simulink model "sl_onelink_control"  (R2017a)
settings: Solver=VariableStepAuto  StartTime=0.0  StopTime=10.0  RelTol=1e-3
libraries: roblocks x2
settings Model: Creator=mkillpack  LastModifiedBy=mkillpack

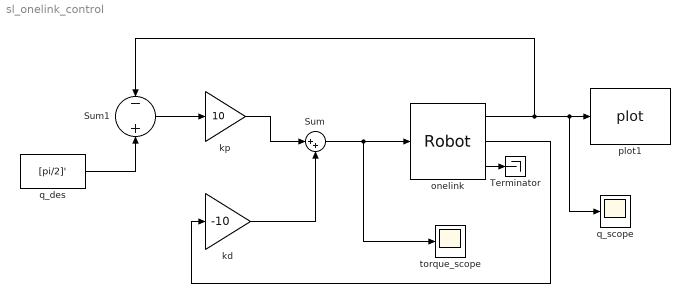
== system sl_onelink_control ==
  Sum : Sum  Inputs=|++
  Sum1 : Sum  Inputs=-|+
  Terminator : Terminator
  kd : Gain  Gain=-10
  kp : Gain  Gain=10
  "onelink " : roblocks/Arm/Robot  robot=onelink  q0=[0]
  plot1 : roblocks/Arm/plot  robot=onelink  fps=10  holdplot=on
  q_des : Constant  Value=[pi/2]'
  q_scope : Scope
  torque_scope : Scope
  wires:
  "onelink "/1 -> Sum1/1, plot1/1, q_scope/1
  Sum1/1 -> kp/1
  kp/1 -> Sum/1
  "onelink "/2 -> kd/1
  kd/1 -> Sum/2
  Sum/1 -> "onelink "/1, torque_scope/1
  q_des/1 -> Sum1/2
  "onelink "/3 -> Terminator/1
